simulink model "acc_with_sensor_copy"  (R2021b)
settings: Solver=FixedStepAuto  StartTime=0.0  StopTime=206  FixedStep=0.0005  RelTol=1e-3
InitFcn:
  | G=9.81;
  | m=1660;
  | rw=0.325;
  | Caf=74070;
  | Car=58525;
  | Iz=2778.5;
  | d = 1.502;
  | lf =1.1135;
  | lr =1.5065;
  | L = 2.62;
  | kph2mps=1/3.6;
values from neighbouring files (symbols this model uses):
  Leftdis_PV_switch = 2    [acc_plot_backup.m]
  s_path = [0 1.10508939428 2.2141958029 3.32141571172 4.42705301151 5.53154548532 6.63517443471 7.73808041313 8.84055018688 9.94289959674 11.0453539299 12.1480581097 ... (1001 elements, 1001x1)]    [200_100radius.mat]    (also in LV_Clothoid_S_Turn_path.mat = [0 0.966832089581 1.93621320584 2.90214024471 3.86476766313 ; NEDC_path.mat = [0 0.414605943146 0.832514087334 1.25401518562 1.68216660344; Straight_East_into_curve.mat = [0 1.65770560069 3.32192925577 4.98420060507 6.64484613518 8; acc_plot_backup.m = Station_HV_m)
  X_path = [0 1.10508939428 2.2141958029 3.32141571172 4.42705301151 5.53154548532 6.63517443471 7.73808041313 8.84055018688 9.94289959674 11.0453539299 12.1480581097 ... (1001 elements, 1001x1)]    [200_100radius.mat]    (also in LV_Clothoid_S_Turn_path.mat = [-10 -9.03316791042 -8.06378679416 -7.09785975529 -6.1352323; NEDC_path.mat = [0 0.414605943146 0.832514087334 1.25401518562 1.68216660344; Straight_East_into_curve.mat = [0 1.65770560069 3.32192925577 4.98420060507 6.64484613518 8; acc_plot_backup.m = X_HV_m)
  Y_path = [0 -1.70364610795e-18 -7.41532896709e-18 1.46822109542e-17 4.74557362791e-17 6.12980216762e-17 9.25043977736e-17 1.24088240159e-16 1.5099156923e-16 1.7058517853e-16 1.90629227614e-16 2.09673434424e-16 ... (1001 elements, 1001x1)]    [200_100radius.mat]    (also in LV_Clothoid_S_Turn_path.mat = [0 -8.46153035536e-19 5.07382551045e-18 2.07356032218e-17 3.; NEDC_path.mat = [0 -3.50680326162e-18 -2.14111304971e-18 3.38197671014e-18 3; Straight_East_into_curve.mat = [0 1.29197709199e-18 2.81882429322e-18 3.49020462564e-17 6.7; acc_plot_backup.m = Y_HV_m)
undefined symbols (not defined in the file or in its folder): C_TICK_TIME_S, Cut_in_Secenary_flg, ENUM_ACCSTATE_DISABLED, ENUM_ACCSTATE_OFF, ENUM_ACCSTATE_STANDBY, FALSE, KVDI_ACCLongPressTime_ms, KVDI_ACCMaxActSpeed_kph, KVDI_ACCSetSpdIntial_kph, KVDI_ACCSpdLargeChange_kph, KVDI_LongPressConTime_ms, ONE_FLOAT, ONE_INT, Path_selector, R, Rw, T, TRUE, UseTTC_switch, ZERO_FLOAT, ZERO_INT
libraries: simulink x15, dspstat3 x4, simulink_extras x2, Solver_SF x1
(part 6 of 8)

== system acc_with_sensor_copy/V_rel Estimation ==
  cut_in_flg : Inport
  a_c : Inport  Port=2
  S_rel : Inport  Port=3
  initial_value : Inport  Port=4
  Add3 : Sum  Inputs=-+
  Delay1 : Delay  DelayLength=1  InitialConditionSource=Input port  SampleTime=0.1
      settings: InputPortMap=u0,p4
  Kalman filter : Subsystem
  sample time : Gain  Gain=1/0.1
  s_rel : Outport
  v_rel : Outport  Port=2
  a_rel : Outport  Port=3
  wires:
  S_rel/1 -> Kalman filter/3(S_rel)
  Kalman filter/1(s_rel) -> s_rel/1
  Add3/1 -> sample time/1
  Delay1/1 -> Add3/1
  a_c/1 -> Delay1/1, Delay1/2, Add3/2
  Kalman filter/2(v_rel) -> v_rel/1
  sample time/1 -> Kalman filter/2(Jerk)  "Jerk"
  Kalman filter/3(a_rel) -> a_rel/1
  initial_value/1 -> Kalman filter/4(initial_value)
  cut_in_flg/1 -> Kalman filter/1(cut_in_flg)

== system acc_with_sensor_copy/acceleration_apr1 ==
  acc_b : Inport
  Abs : Abs
  Constant1 : Constant  Value=0
  Switch : Switch  Criteria=u2 > Threshold  Threshold=0.01
  acc_a : Outport  VectorParamsAs1DForOutWhenUnconnected=off
  wires:
  Switch/1 -> acc_a/1
  acc_b/1 -> Abs/1, Switch/1
  Constant1/1 -> Switch/3
  Abs/1 -> Switch/2

== system acc_with_sensor_copy/acceleration_apr4 ==
  acc_b : Inport
  Abs : Abs
  Constant1 : Constant  Value=0
  Switch : Switch  Criteria=u2 > Threshold  Threshold=0.01
  acc_a : Outport  VectorParamsAs1DForOutWhenUnconnected=off
  wires:
  Abs/1 -> Switch/2
  Constant1/1 -> Switch/3
  acc_b/1 -> Switch/1, Abs/1
  Switch/1 -> acc_a/1

== system acc_with_sensor_copy/cmd_limiter1 ==
  ax_cmd : Inport
  Constant : Constant  Value=0.1  SampleTime=0.1
  Constant1 : Constant  Value=2.5  SampleTime=0.1
  Constant2 : Constant  Value=-2.5  SampleTime=0.1
  Saturation : Saturate  UpperLimit=2  LowerLimit=-2
  rate_limit : Subsystem
  ax_cmd1 : Outport
  wires:
  Constant2/1 -> rate_limit/4(ratelimt_decps)
  Constant1/1 -> rate_limit/3(ratelimt_incps)
  ax_cmd/1 -> Saturation/1
  Constant/1 -> rate_limit/2(Sample_Time)
  rate_limit/1(ax_cmd1) -> ax_cmd1/1
  Saturation/1 -> rate_limit/1(input_raw)

== system acc_with_sensor_copy/cmd_limiter4 ==
  ax_cmd : Inport
  Constant : Constant  Value=0.1  SampleTime=0.1
  Constant1 : Constant  Value=2.5  SampleTime=0.1
  Constant2 : Constant  Value=-2.5  SampleTime=0.1
  Saturation : Saturate  UpperLimit=2  LowerLimit=-2
  rate_limit : Subsystem
  ax_cmd1 : Outport
  wires:
  rate_limit/1(ax_cmd1) -> ax_cmd1/1
  Constant/1 -> rate_limit/2(Sample_Time)
  ax_cmd/1 -> Saturation/1
  Constant1/1 -> rate_limit/3(ratelimt_incps)
  Constant2/1 -> rate_limit/4(ratelimt_decps)
  Saturation/1 -> rate_limit/1(input_raw)

== system acc_with_sensor_copy/divide ==
  dividend : Inport
  divisor : Inport  Port=2
  default_value : Inport  Port=3
  Divide : Product  Inputs=*/
  Interval Test : simulink/Logic and Bit Operations/Interval Test  IntervalClosedRight=on  uplimit=5/3.6  IntervalClosedLeft=on  lowlimit=-1  OutDataTypeStr=boolean
  Logical Operator : Logic  Operator=NOT  Inputs=1  AllPortsSameDT=off  OutDataTypeStr=boolean
  Scope : Scope
  Switch : Switch  Criteria=u2 ~= 0  Threshold=0.5
  quotient : Outport
  wires:
  Logical Operator/1 -> Switch/2
  default_value/1 -> Switch/3  "default_value"
  Interval Test/1 -> Scope/1, Logical Operator/1
  Switch/1 -> quotient/1
  Divide/1 -> Switch/1
  divisor/1 -> Interval Test/1, Divide/2  "divisor"
  dividend/1 -> Divide/1  "dividend"

== system acc_with_sensor_copy/divide1 ==
  dividend : Inport
  divisor : Inport  Port=2
  default_value : Inport  Port=3
  Divide : Product  Inputs=*/
  Interval Test : simulink/Logic and Bit Operations/Interval Test  IntervalClosedRight=on  uplimit=1  IntervalClosedLeft=on  lowlimit=-1  OutDataTypeStr=boolean
  Logical Operator : Logic  Operator=NOT  Inputs=1  AllPortsSameDT=off  OutDataTypeStr=boolean
  Scope : Scope
  Switch : Switch  Criteria=u2 ~= 0  Threshold=0.5
  quotient : Outport
  wires:
  Logical Operator/1 -> Switch/2
  default_value/1 -> Switch/3  "default_value"
  Interval Test/1 -> Scope/1, Logical Operator/1
  Switch/1 -> quotient/1
  Divide/1 -> Switch/1
  divisor/1 -> Interval Test/1, Divide/2  "divisor"
  dividend/1 -> Divide/1  "dividend"

== system acc_with_sensor_copy/divide2 ==
  dividend : Inport
  divisor : Inport  Port=2
  default_value : Inport  Port=3
  Divide : Product  Inputs=*/
  Interval Test : simulink/Logic and Bit Operations/Interval Test  IntervalClosedRight=on  uplimit=15/3.6  IntervalClosedLeft=on  lowlimit=-1  OutDataTypeStr=boolean
  Logical Operator : Logic  Operator=NOT  Inputs=1  AllPortsSameDT=off  OutDataTypeStr=boolean
  Scope : Scope
  Switch : Switch  Criteria=u2 ~= 0  Threshold=0.5
  quotient : Outport
  wires:
  dividend/1 -> Divide/1  "dividend"
  divisor/1 -> Divide/2, Interval Test/1  "divisor"
  Divide/1 -> Switch/1
  Switch/1 -> quotient/1
  Interval Test/1 -> Logical Operator/1, Scope/1
  default_value/1 -> Switch/3  "default_value"
  Logical Operator/1 -> Switch/2

== system acc_with_sensor_copy/divide3 ==
  dividend : Inport
  divisor : Inport  Port=2
  default_value : Inport  Port=3
  Divide : Product  Inputs=*/
  Interval Test : simulink/Logic and Bit Operations/Interval Test  IntervalClosedRight=on  uplimit=-0.1  IntervalClosedLeft=on  lowlimit=-inf  OutDataTypeStr=boolean
  Logical Operator : Logic  Operator=NOT  Inputs=1  AllPortsSameDT=off  OutDataTypeStr=boolean
  Scope : Scope
  Switch : Switch  Criteria=u2 ~= 0  Threshold=0.5
  quotient : Outport
  wires:
  dividend/1 -> Divide/1  "dividend"
  divisor/1 -> Divide/2, Interval Test/1  "divisor"
  Divide/1 -> Switch/1
  Switch/1 -> quotient/1
  Interval Test/1 -> Logical Operator/1, Scope/1
  default_value/1 -> Switch/3  "default_value"
  Logical Operator/1 -> Switch/2

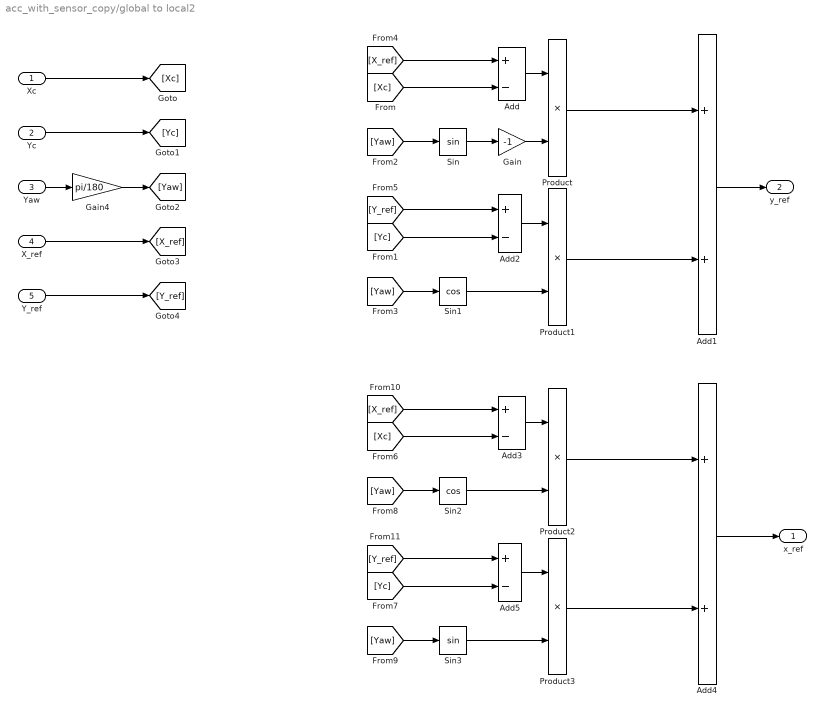
== system acc_with_sensor_copy/global to local2 ==
  Xc : Inport
  Yc : Inport  Port=2
  Yaw : Inport  Port=3
  X_ref : Inport  Port=4
  Y_ref : Inport  Port=5
  Add{,2..3,5} (4 alike) : Sum  Inputs=+-
  Add1 : Sum
  Add4 : Sum
  Gain : Gain  Gain=-1
  Gain4 : Gain  Gain=pi/180
  Product{,1..3} (4 alike) : Product
  Sin : Trigonometry
  Sin1 : Trigonometry  Operator=cos
  Sin2 : Trigonometry  Operator=cos
  Sin3 : Trigonometry
  x_ref : Outport
  y_ref : Outport  Port=2
  wires:
  [X_ref] -> Add3/1
  [Y_ref] -> Add5/1
  Sin2/1 -> Product2/2
  Add3/1 -> Product2/1
  Product2/1 -> Add4/1
  Sin3/1 -> Product3/2
  Add5/1 -> Product3/1
  Product3/1 -> Add4/2
  Add4/1 -> x_ref/1
  [Yaw] -> Sin2/1
  [Yc] -> Add5/2
  [Xc] -> Add3/2
  [Yaw] -> Sin3/1
  Gain4/1 -> [Yaw]
  Y_ref/1 -> [Y_ref]
  X_ref/1 -> [X_ref]
  [Yaw] -> Sin1/1
  Yaw/1 -> Gain4/1
  Yc/1 -> [Yc]
  Xc/1 -> [Xc]
  [Xc] -> Add/2
  [Yc] -> Add2/2
  [Yaw] -> Sin/1
  Add1/1 -> y_ref/1
  Product1/1 -> Add1/2
  Add2/1 -> Product1/1
  Sin1/1 -> Product1/2
  Product/1 -> Add1/1
  Add/1 -> Product/1
  Gain/1 -> Product/2
  Sin/1 -> Gain/1
  [Y_ref] -> Add2/1
  [X_ref] -> Add/1

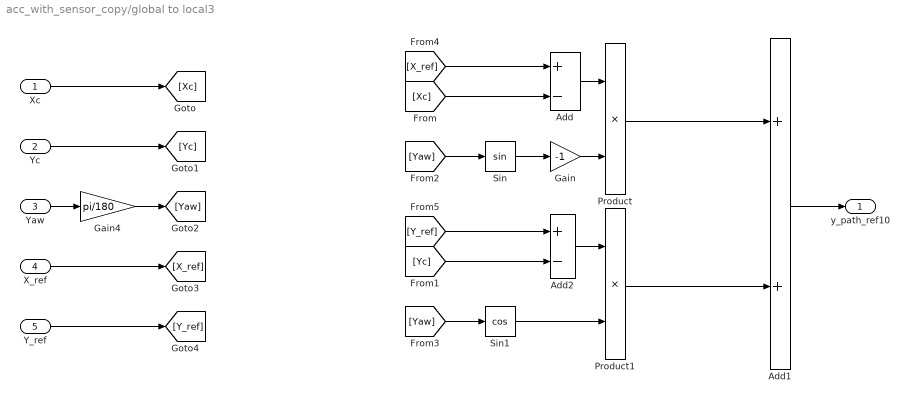
== system acc_with_sensor_copy/global to local3 ==
  Xc : Inport
  Yc : Inport  Port=2
  Yaw : Inport  Port=3
  X_ref : Inport  Port=4
  Y_ref : Inport  Port=5
  Add : Sum  Inputs=+-
  Add1 : Sum
  Add2 : Sum  Inputs=+-
  Gain : Gain  Gain=-1
  Gain4 : Gain  Gain=pi/180
  Product : Product
  Product1 : Product
  Sin : Trigonometry
  Sin1 : Trigonometry  Operator=cos
  y_path_ref10 : Outport
  wires:
  Gain4/1 -> [Yaw]
  Y_ref/1 -> [Y_ref]
  X_ref/1 -> [X_ref]
  [Yaw] -> Sin1/1
  Yaw/1 -> Gain4/1
  Yc/1 -> [Yc]
  Xc/1 -> [Xc]
  [Xc] -> Add/2
  [Yc] -> Add2/2
  [Yaw] -> Sin/1
  Add1/1 -> y_path_ref10/1
  Product1/1 -> Add1/2
  Add2/1 -> Product1/1
  Sin1/1 -> Product1/2
  Product/1 -> Add1/1
  Add/1 -> Product/1
  Gain/1 -> Product/2
  Sin/1 -> Gain/1
  [Y_ref] -> Add2/1
  [X_ref] -> Add/1

== system acc_with_sensor_copy/preview ==
  In1 : Inport
  In2 : Inport  Port=2
  Add9 : Sum
  Constant20 : Constant  Value=s_path
  Constant21 : Constant  Value=X_path
  Constant22 : Constant  Value=s_path
  Constant23 : Constant  Value=Y_path
  Constant49 : Constant  Value=[1:10]'
  Constant51 : Constant  Value=0.1
  Demux4 : Demux  Outputs=[1 9]
  Demux5 : Demux  Outputs=[1 9]
  Lookup Table Dynamic : simulink/Lookup Tables/Lookup Table Dynamic  LookUpMeth=Interpolation-Use End Values  OutDataType=fixdt('double')  OutScaling=[]  OutputDataTypeScalingMode=Specify via dialog  OutDataTypeStr=double  DoSatur=off
  Lookup Table Dynamic1 : simulink/Lookup Tables/Lookup Table Dynamic  LookUpMeth=Interpolation-Use End Values  OutDataType=fixdt('double')  OutScaling=[]  OutputDataTypeScalingMode=Specify via dialog  OutDataTypeStr=double  DoSatur=off
  Product1 : Product
  Product10 : Product
  Scope7 : Scope
  Terminator : Terminator
  Terminator1 : Terminator
  To Workspace27 : ToWorkspace  VariableName=X_ref  SampleTime=-1
  To Workspace28 : ToWorkspace  VariableName=Y_ref  SampleTime=-1
  X_ref : Outport
  Y_ref : Outport  Port=2
  wires:
  Constant23/1 -> Lookup Table Dynamic1/3
  Product10/1 -> Add9/2
  Product1/1 -> Product10/2
  Constant22/1 -> Lookup Table Dynamic1/2
  Constant20/1 -> Lookup Table Dynamic/2
  Constant21/1 -> Lookup Table Dynamic/3
  Lookup Table Dynamic1/1 -> Y_ref/1, Demux5/1
  Demux5/1 -> To Workspace28/1
  In1/1 -> Add9/1
  Lookup Table Dynamic/1 -> X_ref/1, Demux4/1
  In2/1 -> Product10/1
  Constant51/1 -> Product1/2
  Add9/1 -> Lookup Table Dynamic1/1, Scope7/1, Lookup Table Dynamic/1
  Constant49/1 -> Product1/1
  Demux4/1 -> To Workspace27/1
  Demux5/2 -> Terminator1/1
  Demux4/2 -> Terminator/1

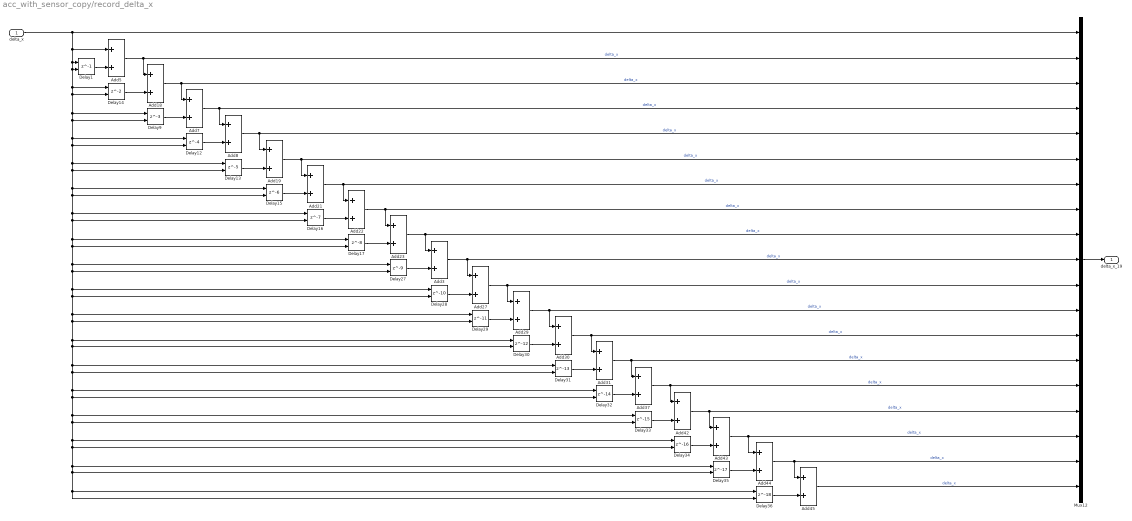
== system acc_with_sensor_copy/record_delta_x ==
  delta_x : Inport
  Add{3,5,7..8,18..19,21..23,27,29..31,37,42..45} (18 alike) : Sum
  Delay1 : Delay  DelayLength=1  InitialConditionSource=Input port
      settings: InputPortMap=u0,p4
  Delay12 : Delay  DelayLength=4  InitialConditionSource=Input port
      settings: InputPortMap=u0,p4
  Delay13 : Delay  DelayLength=5  InitialConditionSource=Input port
      settings: InputPortMap=u0,p4
  Delay14 : Delay  InitialConditionSource=Input port
      settings: InputPortMap=u0,p4
  Delay15 : Delay  DelayLength=6  InitialConditionSource=Input port
      settings: InputPortMap=u0,p4
  Delay16 : Delay  DelayLength=7  InitialConditionSource=Input port
      settings: InputPortMap=u0,p4
  Delay17 : Delay  DelayLength=8  InitialConditionSource=Input port
      settings: InputPortMap=u0,p4
  Delay27 : Delay  DelayLength=9  InitialConditionSource=Input port
      settings: InputPortMap=u0,p4
  Delay28 : Delay  DelayLength=10  InitialConditionSource=Input port
      settings: InputPortMap=u0,p4
  Delay29 : Delay  DelayLength=11  InitialConditionSource=Input port
      settings: InputPortMap=u0,p4
  Delay30 : Delay  DelayLength=12  InitialConditionSource=Input port
      settings: InputPortMap=u0,p4
  Delay31 : Delay  DelayLength=13  InitialConditionSource=Input port
      settings: InputPortMap=u0,p4
  Delay32 : Delay  DelayLength=14  InitialConditionSource=Input port
      settings: InputPortMap=u0,p4
  Delay33 : Delay  DelayLength=15  InitialConditionSource=Input port
      settings: InputPortMap=u0,p4
  Delay34 : Delay  DelayLength=16  InitialConditionSource=Input port
      settings: InputPortMap=u0,p4
  Delay35 : Delay  DelayLength=17  InitialConditionSource=Input port
      settings: InputPortMap=u0,p4
  Delay36 : Delay  DelayLength=18  InitialConditionSource=Input port
      settings: InputPortMap=u0,p4
  Delay9 : Delay  DelayLength=3  InitialConditionSource=Input port
      settings: InputPortMap=u0,p4
  Mux12 : Mux  Inputs=19
  delta_x_19 : Outport
  wires:
  Add19/1 -> Mux12/6, Add21/1  "delta_x"
  Delay13/1 -> Add19/2
  Add44/1 -> Add45/1, Mux12/18  "delta_x"
  delta_x/1 -> Mux12/1, Delay14/2, Delay9/1, Delay15/1, Delay27/2, Delay28/1, Delay30/2, Delay31/1, Delay32/1, Delay33/1, Delay33/2, Delay34/1, Delay35/1, Delay36/1, Delay36/2, Delay35/2, Delay34/2, Delay32/2, Delay31/2, Delay30/1, Delay29/2, Delay29/1, Delay28/2, Delay27/1, Delay17/2, Delay17/1, Delay16/2, Delay16/1, Delay15/2, Delay13/2, Delay13/1, Delay12/2, Delay12/1, Delay9/2, Delay14/1, Delay1/2, Delay1/1, Add5/1
  Add29/1 -> Mux12/12, Add30/1  "delta_x"
  Add5/1 -> Mux12/2, Add18/1  "delta_x"
  Add18/1 -> Mux12/3, Add7/1  "delta_x"
  Delay29/1 -> Add29/2
  Delay1/1 -> Add5/2
  Add31/1 -> Mux12/14, Add37/1  "delta_x"
  Delay33/1 -> Add42/2
  Add23/1 -> Mux12/9, Add3/1  "delta_x"
  Delay9/1 -> Add7/2
  Add42/1 -> Add43/1, Mux12/16  "delta_x"
  Mux12/1 -> delta_x_19/1
  Delay14/1 -> Add18/2
  Add21/1 -> Mux12/7, Add22/1  "delta_x"
  Add30/1 -> Mux12/13, Add31/1  "delta_x"
  Delay34/1 -> Add43/2
  Delay17/1 -> Add23/2
  Delay27/1 -> Add3/2
  Add45/1 -> Mux12/19  "delta_x"
  Delay31/1 -> Add31/2
  Add43/1 -> Add44/1, Mux12/17  "delta_x"
  Delay15/1 -> Add21/2
  Add8/1 -> Mux12/5, Add19/1  "delta_x"
  Delay32/1 -> Add37/2
  Delay35/1 -> Add44/2
  Delay36/1 -> Add45/2
  Add27/1 -> Mux12/11, Add29/1  "delta_x"
  Add3/1 -> Mux12/10, Add27/1  "delta_x"
  Delay28/1 -> Add27/2
  Delay16/1 -> Add22/2
  Add22/1 -> Mux12/8, Add23/1  "delta_x"
  Delay30/1 -> Add30/2
  Add37/1 -> Mux12/15, Add42/1  "delta_x"
  Delay12/1 -> Add8/2
  Add7/1 -> Mux12/4, Add8/1  "delta_x"

== system acc_with_sensor_copy/record_delta_yaw ==
  delta_yaw : Inport
  Add78 : Sum  Inputs=+-
  Delay68 : Delay  DelayLength=1  InitialConditionSource=Input port
      settings: InputPortMap=u0,p4
  Delay69 : Delay  InitialConditionSource=Input port
      settings: InputPortMap=u0,p4
  Delay70 : Delay  DelayLength=3  InitialConditionSource=Input port
      settings: InputPortMap=u0,p4
  Delay71 : Delay  DelayLength=4  InitialConditionSource=Input port
      settings: InputPortMap=u0,p4
  Delay72 : Delay  DelayLength=5  InitialConditionSource=Input port
      settings: InputPortMap=u0,p4
  Delay73 : Delay  DelayLength=6  InitialConditionSource=Input port
      settings: InputPortMap=u0,p4
  Delay74 : Delay  DelayLength=7  InitialConditionSource=Input port
      settings: InputPortMap=u0,p4
  Delay75 : Delay  DelayLength=8  InitialConditionSource=Input port
      settings: InputPortMap=u0,p4
  Delay76 : Delay  DelayLength=9  InitialConditionSource=Input port
      settings: InputPortMap=u0,p4
  Delay77 : Delay  DelayLength=10  InitialConditionSource=Input port
      settings: InputPortMap=u0,p4
  Delay78 : Delay  DelayLength=11  InitialConditionSource=Input port
      settings: InputPortMap=u0,p4
  Delay79 : Delay  DelayLength=12  InitialConditionSource=Input port
      settings: InputPortMap=u0,p4
  Delay80 : Delay  DelayLength=13  InitialConditionSource=Input port
      settings: InputPortMap=u0,p4
  Delay81 : Delay  DelayLength=14  InitialConditionSource=Input port
      settings: InputPortMap=u0,p4
  Delay82 : Delay  DelayLength=15  InitialConditionSource=Input port
      settings: InputPortMap=u0,p4
  Delay83 : Delay  DelayLength=16  InitialConditionSource=Input port
      settings: InputPortMap=u0,p4
  Delay84 : Delay  DelayLength=17  InitialConditionSource=Input port
      settings: InputPortMap=u0,p4
  Delay85 : Delay  DelayLength=18  InitialConditionSource=Input port
      settings: InputPortMap=u0,p4
  Delay86 : Delay  DelayLength=19  InitialConditionSource=Input port
      settings: InputPortMap=u0,p4
  Mux18 : Mux  Inputs=19
  delta_yaw_19 : Outport
  wires:
  Delay84/1 -> Mux18/17
  Delay72/1 -> Mux18/5
  Delay73/1 -> Mux18/6
  Delay78/1 -> Mux18/11
  Delay71/1 -> Mux18/4
  Delay68/1 -> Mux18/1
  Delay76/1 -> Mux18/9
  delta_yaw/1 -> Delay68/1, Delay68/2, Delay86/2, Delay86/1, Delay85/2, Delay85/1, Delay84/2, Delay84/1, Delay83/2, Delay83/1, Delay82/2, Delay82/1, Delay81/2, Delay81/1, Delay80/2, Delay80/1, Delay79/2, Delay79/1, Delay78/2, Delay78/1, Delay77/2, Delay77/1, Delay76/2, Delay76/1, Delay75/2, Delay75/1, Delay74/2, Delay74/1, Delay73/2, Delay73/1, Delay72/2, Delay72/1, Delay71/2, Delay71/1, Delay70/2, Delay70/1, Delay69/2, Delay69/1, Add78/1
  Delay81/1 -> Mux18/14
  Delay75/1 -> Mux18/8
  Delay80/1 -> Mux18/13
  Delay86/1 -> Mux18/19
  Delay82/1 -> Mux18/15
  Delay69/1 -> Mux18/2
  Delay70/1 -> Mux18/3
  Delay74/1 -> Mux18/7
  Mux18/1 -> Add78/2
  Delay77/1 -> Mux18/10
  Add78/1 -> delta_yaw_19/1
  Delay85/1 -> Mux18/18
  Delay79/1 -> Mux18/12
  Delay83/1 -> Mux18/16

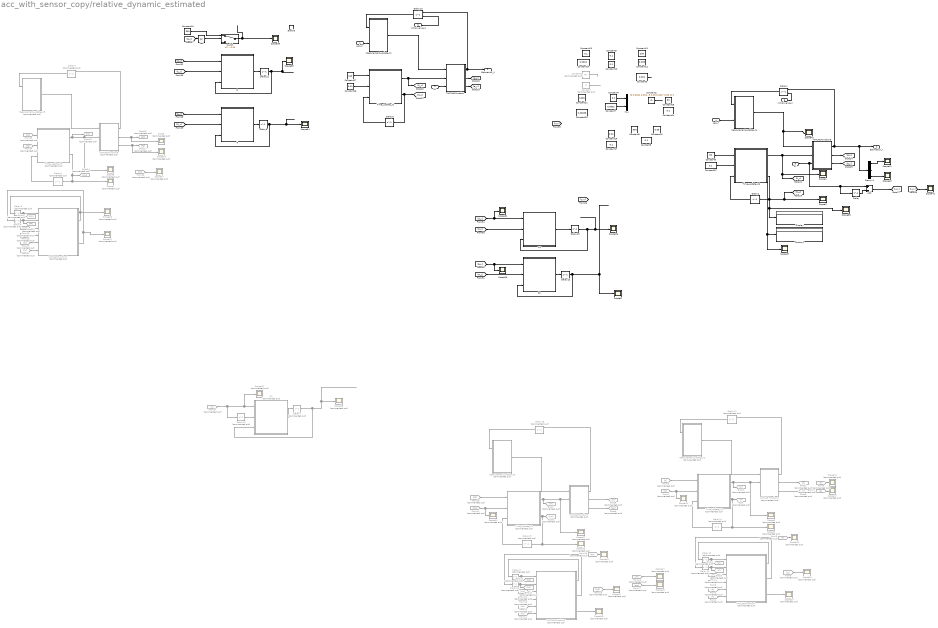
== system acc_with_sensor_copy/relative_dynamic_estimated ==
  Jerk_X : Inport
  RX : Inport  Port=2
  Initial_value_X : Inport  Port=3
  Jerk_Y : Inport  Port=4
  RY : Inport  Port=5
  Initial_value_Y : Inport  Port=6
  Enable : EnablePort
  Abs : Abs
  Add : Sum  Inputs=+-
  Constant : Constant  Commented=on  Value=R
  Constant1 : Constant  Commented=on  Value=Rw
  Constant{4..5,9..10,13,17,22,24} (8 alike) : Constant  Value=0.1
  Constant11 : Constant  Value=200
  Constant12 : Constant  Value=0.005
  Constant14 : Constant  Value=0.0001
  Constant15 : Constant  Value=0.05
  Constant16 : Constant  Value=300
  Constant19 : Constant  Value=0.01
  Constant2 : Constant  Value=[0 0.0001 0.0017;0.0001 0.0025 0.05;0.0017 0.05 1]*1
  Constant20 : Constant  Value=0.00005
  Constant21 : Constant  Value=1000
  Constant25 : Constant  Value=50
  Constant26 : Constant  Value=0.01
  Constant27 : Constant  Value=100
  Constant3 : Constant  Value=0.001
  Constant6 : Constant  Value=50
  Constant7 : Constant  Value=0.0001
  Constant8 : Constant  Value=500
  Delay : Delay  DelayLength=1
  Delay1 : Delay  DelayLength=1  InitialConditionSource=Input port  InitialCondition=[0;0;0]  SampleTime=T
      settings: InputPortMap=u0,p4
  Delay10 : Delay  DelayLength=1  InitialConditionSource=Input port  InitialCondition=[0;0;0]  SampleTime=T
      settings: InputPortMap=u0,p4
  Delay11 : Delay  Commented=on  DelayLength=1  InitialConditionSource=Input port  InitialCondition=[0;0;0]  SampleTime=T
      settings: InputPortMap=u0,p4
  Delay12 : Delay  Commented=on  DelayLength=1  InitialCondition=[0 0 0;0 0 0.004;0 0.004 0.8]*0.001  SampleTime=T
  Delay13 : Delay  Commented=on  DelayLength=1  InitialCondition=0.001  SampleTime=T
  Delay14 : Delay  Commented=on  DelayLength=1  InitialCondition=[1 0 0;0 1 0;0 0 1]  SampleTime=T
  Delay15 : Delay  Commented=on  DelayLength=1  InitialConditionSource=Input port  InitialCondition=[0;0;0]  SampleTime=T
      settings: InputPortMap=u0,p4
  Delay16 : Delay  Commented=on  DelayLength=1  InitialCondition=0
  Delay17 : Delay  Commented=on  DelayLength=1  InitialCondition=[0 0 0;0 0 0.004;0 0.004 0.8]*0.01  SampleTime=T
  Delay18 : Delay  Commented=on  DelayLength=1  InitialCondition=0.001  SampleTime=T
  Delay19 : Delay  Commented=on  DelayLength=1  InitialCondition=[1 0 0;0 1 0;0 0 1]  SampleTime=T
  Delay2 : Delay  DelayLength=1  InitialCondition=[1 0 0;0 1 0;0 0 1]  SampleTime=T
  Delay21 : Delay  DelayLength=1  InitialCondition=[0 0.0001 0.0017;0.0001 0.0025 0.05;0.0017 0.05 1]
  Delay22 : Delay  DelayLength=1  InitialCondition=0.001
  Delay23 : Delay  DelayLength=1  InitialCondition=[0 0.0001 0.0017;0.0001 0.0025 0.05;0.0017 0.05 1]*1e-5
  Delay3 : Delay  Commented=on  DelayLength=1  InitialCondition=[0 0 0;0 0 0.003;0 0.003 0.005]  SampleTime=T
  Delay4 : Delay  Commented=on  DelayLength=1  InitialConditionSource=Input port  InitialCondition=[0;0;0]  SampleTime=T
      settings: InputPortMap=u0,p4
  Delay5 : Delay  Commented=on  DelayLength=1  InitialCondition=0.001  SampleTime=T
  Delay6 : Delay  Commented=on  DelayLength=1  InitialCondition=[1 0 0;0 1 0;0 0 1]  SampleTime=T
  Delay7 : Delay  Commented=on  DelayLength=1  InitialCondition=0.1
  Delay8 : Delay  DelayLength=1  InitialCondition=0.1
  Delay9 : Delay  DelayLength=1  InitialCondition=[1 0 0;0 1 0;0 0 1]  SampleTime=T
  Demux1 : Demux  Outputs=3
  Display : Display
  Display1 : Display
  From : From  Commented=on  GotoTag=M
  From1 : From  Commented=on  GotoTag=K
  From10 : From  Commented=on  GotoTag=MM
  From11 : From  Commented=on  GotoTag=KK
  From12 : From  Commented=on  GotoTag=dd
  From13 : From  Commented=on  GotoTag=ee
  From14 : From  Commented=on  GotoTag=QQ
  From15 : From  Commented=on  GotoTag=RR
  From16 : From  Commented=on  GotoTag=dd
  From17 : From  Commented=on  GotoTag=ee
  From18 : From  Commented=on  GotoTag=RR
  From19 : From  Commented=on  GotoTag=QQ
  From2 : From  Commented=on  GotoTag=d
  From20 : From  Commented=on  GotoTag=MM
  From21 : From  Commented=on  GotoTag=KK
  From22 : From  Commented=on  GotoTag=dd
  From23 : From  Commented=on  GotoTag=ee
  From24 : From  Commented=on  GotoTag=QQ
  From25 : From  Commented=on  GotoTag=RR
  From26 : From  Commented=on  GotoTag=KK
  From27 : From  Commented=on  GotoTag=d
  From3 : From  Commented=on  GotoTag=e
  From4 : From  Commented=on  GotoTag=Q
  From5 : From  Commented=on  GotoTag=R
  From6 : From  Commented=on  GotoTag=d
  From7 : From  Commented=on  GotoTag=e
  From8 : From  Commented=on  GotoTag=R
  From9 : From  Commented=on  GotoTag=Q
  Goto : Goto  Commented=on  GotoTag=M
  Goto1 : Goto  Commented=on  GotoTag=K
  Goto10 : Goto  Commented=on  GotoTag=QQ
  Goto11 : Goto  Commented=on  GotoTag=RR
  Goto12 : Goto  Commented=on  GotoTag=QQ
  Goto13 : Goto  Commented=on  GotoTag=RR
  Goto14 : Goto  Commented=on  GotoTag=MM
  Goto15 : Goto  Commented=on  GotoTag=KK
  Goto16 : Goto  Commented=on  GotoTag=dd
  Goto17 : Goto  Commented=on  GotoTag=ee
  Goto2 : Goto  Commented=on  GotoTag=d
  Goto3 : Goto  Commented=on  GotoTag=e
  Goto4 : Goto  Commented=on  GotoTag=Q
  Goto5 : Goto  Commented=on  GotoTag=R
  Goto6 : Goto  Commented=on  GotoTag=MM
  Goto7 : Goto  Commented=on  GotoTag=KK
  Goto8 : Goto  Commented=on  GotoTag=dd
  Goto9 : Goto  Commented=on  GotoTag=ee
  MATLAB Function : MATLAB Function  TreatAsAtomicUnit=on
  MATLAB Function1 : MATLAB Function  Commented=on  TreatAsAtomicUnit=on
  MATLAB Function2 : MATLAB Function  Commented=on  TreatAsAtomicUnit=on
  MATLAB Function3 : MATLAB Function  Commented=on  TreatAsAtomicUnit=on
  MATLAB Function4 : MATLAB Function  Commented=on  TreatAsAtomicUnit=on
  MATLAB Function5 : MATLAB Function  TreatAsAtomicUnit=on
  MATLAB Function6 : MATLAB Function  Commented=on  TreatAsAtomicUnit=on
  MATLAB Function7 : MATLAB Function  Commented=on  TreatAsAtomicUnit=on
  Measurement_update_X1 : MATLAB Function  TreatAsAtomicUnit=on
  Measurement_update_X2 : MATLAB Function  Commented=on  TreatAsAtomicUnit=on
  Measurement_update_X3 : MATLAB Function  Commented=on  TreatAsAtomicUnit=on
  Measurement_update_X4 : MATLAB Function  TreatAsAtomicUnit=on
  Measurement_update_X5 : MATLAB Function  Commented=on  TreatAsAtomicUnit=on
  Mux : Mux  Inputs=2
  Q : MATLAB Function  TreatAsAtomicUnit=on
  Q1 : MATLAB Function  Commented=on  TreatAsAtomicUnit=on
  Q2 : MATLAB Function  TreatAsAtomicUnit=on
  R : MATLAB Function  TreatAsAtomicUnit=on
  R2 : MATLAB Function  TreatAsAtomicUnit=on
  Scope{,6..28,30} (25 alike) : Scope  Commented=on
  Scope{1..2,5,29,31,34..43} (15 alike) : Scope
  Switch : Switch  Criteria=u2 > Threshold  Threshold=0.04
  Time_update_X1 : MATLAB Function  TreatAsAtomicUnit=on
  Time_update_X2 : MATLAB Function  Commented=on  TreatAsAtomicUnit=on
  Time_update_X3 : MATLAB Function  Commented=on  TreatAsAtomicUnit=on
  Time_update_X5 : MATLAB Function  Commented=on  TreatAsAtomicUnit=on
  Time_update_X6 : MATLAB Function  TreatAsAtomicUnit=on
  Estimation_X : Outport  VectorParamsAs1DForOutWhenUnconnected=off
  Estimation_Y : Outport  Port=2  VectorParamsAs1DForOutWhenUnconnected=off
  wires:
  MATLAB Function/3(e) -> [e_x]
  MATLAB Function/2(d) -> [d_x]
  Constant27/1 -> Time_update_X1/1(Q)
  Constant26/1 -> Time_update_X1/2(R)
  Abs/1 -> Switch/2
  [d_x] -> Abs/1
  Constant16/1 -> Switch/1
  Switch/1 -> Scope39/1
  Constant22/1 -> Time_update_X6/2(R)
  Constant6/1 -> Time_update_X6/1(Q)
  Demux1/3 -> Scope43/1
  Demux1/1 -> Scope42/1
  [yyy] -> Scope41/1
  Delay/1 -> Add/2
  Add/1 -> [yyy]
  Delay22/1 -> Scope5/1, R2/3(R1)
  Constant7/1 -> Mux/2
  Constant4/1 -> Mux/1
  Demux1/2 -> ?
  Delay23/1 -> Scope36/1, Q2/3(Q1)
  Time_update_X6/2(P) -> Display1/1, Scope37/1
  Constant3/1 -> ?
  Constant2/1 -> ?
  Q2/1(Q) -> Delay23/1
  Constant1/1 -> ?
  Constant/1 -> ?
  MATLAB Function5/3(e) -> [e_y]
  MATLAB Function5/2(d) -> [d_y]
  [d_y] -> Q2/1(d), Scope31/1
  [K_y] -> Q2/2(K)
  R2/1(R) -> Delay22/1
  [M_y] -> R2/2(M)
  [e_y] -> R2/1(e), Scope29/1
  Q1/1(Rw) -> Delay7/1
  From27/1 -> Q1/1(d), Scope30/1, Delay16/1
  Delay7/1 -> Scope28/1, Q1/3(Rw1)
  Delay16/1 -> Q1/2(dx)
  Delay21/1 -> Q/3(Q1), Scope35/1
  Q/1(Q) -> Delay21/1
  [K_x] -> Q/2(K)
  [d_x] -> Q/1(d)
  [M_x] -> R/2(M)
  R/1(R) -> Delay8/1
  [e_x] -> R/1(e)
  Delay8/1 -> R/3(R1), Scope34/1
  RX/1 -> MATLAB Function/3(y)
  From26/1 -> Scope27/1
  Initial_value_X/1 -> Delay10/2
  Delay4/1 -> Measurement_update_X5/1(X_e)
  MATLAB Function6/1(X_e) -> Delay4/1
  Measurement_update_X5/1(X_b) -> MATLAB Function6/1(X_b)
  Time_update_X5/2(M2) -> Scope7/1, Delay6/1, Goto14/1
  From22/1 -> MATLAB Function7/5(d)
  Delay6/1 -> Time_update_X5/3(M)
  Time_update_X5/1(K) -> MATLAB Function6/2(K), Scope6/1, Goto15/1
  From21/1 -> MATLAB Function7/6(K)
  From20/1 -> MATLAB Function7/3(M)
  MATLAB Function7/2(R2) -> Delay5/1, Scope26/1
  MATLAB Function6/3(e) -> Goto17/1, Scope24/1
  From24/1 -> Time_update_X5/2(Q)
  From25/1 -> Time_update_X5/1(R)
  MATLAB Function7/1(Q2) -> Scope25/1, Delay3/1
  From23/1 -> MATLAB Function7/4(e)
  Delay5/1 -> Goto13/1, MATLAB Function7/2(R)
  Delay3/1 -> Goto12/1, MATLAB Function7/1(Q)
  MATLAB Function6/2(d) -> Goto16/1, Scope/1
  RY/1 -> MATLAB Function5/3(y), Delay/1, Add/1
  Initial_value_Y/1 -> Delay1/2
  Measurement_update_X4/1(X_b) -> MATLAB Function5/1(X_b), Scope40/1
  MATLAB Function5/1(X_e) -> Delay1/1, Estimation_Y/1, Demux1/1
  Delay1/1 -> Measurement_update_X4/1(X_e)
  Time_update_X6/1(K) -> Scope1/1, [K_y], MATLAB Function5/2(K)
  Time_update_X6/3(M2) -> Delay2/1, Scope2/1, [M_y], Display/1, Scope38/1
  Delay2/1 -> Time_update_X6/3(M)
  Jerk_Y/1 -> Measurement_update_X4/2(u)
  Jerk_X/1 -> Measurement_update_X1/2(u)
  MATLAB Function3/2(d) -> Goto8/1
  Delay17/1 -> MATLAB Function4/1(Q), Goto10/1
  Time_update_X3/1(K) -> MATLAB Function3/2(K), Scope22/1, Goto7/1
  From13/1 -> MATLAB Function4/4(e)
  From15/1 -> Time_update_X3/1(R)
  From19/1 -> Scope21/1
  MATLAB Function4/1(Q2) -> Delay17/1
  Delay18/1 -> MATLAB Function4/2(R), Goto11/1
  From10/1 -> MATLAB Function4/3(M)
  MATLAB Function4/2(R2) -> Delay18/1
  Delay15/1 -> Measurement_update_X3/1(X_e)
  From11/1 -> MATLAB Function4/6(K)
  Delay19/1 -> Time_update_X3/3(M)
  From12/1 -> MATLAB Function4/5(d)
  From17/1 -> Scope18/1
  From18/1 -> Scope19/1
  From16/1 -> Scope17/1
  MATLAB Function3/3(e) -> Goto9/1
  Time_update_X3/2(M2) -> Goto6/1, Delay19/1, Scope23/1
  Measurement_update_X3/1(X_b) -> MATLAB Function3/1(X_b)
  From14/1 -> Time_update_X3/2(Q), Scope16/1
  MATLAB Function3/1(X_e) -> Delay15/1
  MATLAB Function4/3(G) -> Scope20/1
  From9/1 -> Scope15/1
  MATLAB Function2/3(G) -> Scope14/1
  From8/1 -> Scope13/1
  From7/1 -> Scope12/1
  From6/1 -> Scope11/1
  From4/1 -> Time_update_X2/2(Q), Scope10/1
  MATLAB Function2/1(Q2) -> Delay12/1
  Time_update_X2/2(M2) -> Goto/1, Delay14/1, Scope9/1
  From1/1 -> MATLAB Function2/6(K)
  Delay13/1 -> MATLAB Function2/2(R), Goto5/1
  Delay14/1 -> Time_update_X2/3(M)
  Time_update_X2/1(K) -> MATLAB Function1/2(K), Scope8/1, Goto1/1
  Delay11/1 -> Measurement_update_X2/1(X_e)
  Measurement_update_X2/1(X_b) -> MATLAB Function1/1(X_b)
  MATLAB Function1/1(X_e) -> Delay11/1
  MATLAB Function1/2(d) -> Goto2/1
  From2/1 -> MATLAB Function2/5(d)
  From5/1 -> Time_update_X2/1(R)
  MATLAB Function1/3(e) -> Goto3/1
  MATLAB Function2/2(R2) -> Delay13/1
  From/1 -> MATLAB Function2/3(M)
  From3/1 -> MATLAB Function2/4(e)
  Delay12/1 -> MATLAB Function2/1(Q), Goto4/1
  MATLAB Function/1(X_e) -> Delay10/1, Estimation_X/1
  Time_update_X1/2(M2) -> Delay9/1, [M_x]
  Measurement_update_X1/1(X_b) -> MATLAB Function/1(X_b)
  Delay9/1 -> Time_update_X1/3(M)
  Delay10/1 -> Measurement_update_X1/1(X_e)
  Time_update_X1/1(K) -> MATLAB Function/2(K), [K_x]

== system acc_with_sensor_copy/rolling_avg ==
  note: new_average = [ (sample_interval)/(sample_interval + time_constant) ] * (new_value - old_ave) + old_ave
  note: - (FK_TMR/TC)
      |                                    f  =  1  -  e
      |
      |       Where "f" is called the filter constant in the difference equation:
      |
      |                    new_average = f * new_value + (1 - f) * old_average
  note: Using the first two terms of the series expansion:
      |
      |                     x                     x2
      |                                e   =  1  +  x  +  --  + ......
      |                                           2!
      |
      |       Simplifying, the exponential "f" becomes:
      |
      |                  - (FK_TMR/TC)              1
      |           f  =  1  -  e                    =  1  -  -------------  =  . . .
      |                                                    (FK_TMR/TC)
      |                           e
      |
      |                              1                      1
      |          f  =  1  -  ---------------------------------  =    ------------------- .
      |                                  1 + (FK_TMR / TC)       1 + (TC / FK_TMR)
  new_value : Inport
  old_ave : Inport  Port=2
  delta_t : Inport  Port=3
  tc : Inport  Port=4
  Divide : Product  Inputs=*/
  IC : UnitDelay  Tag=struct('comment',struct('text','','placement',1),'logdata',struct('maxnumvals',inf,'plotchannels',[],'stepsize',0,'downsampling',1,'loggingmode',3,'channels',1),'output',struct('width',1,'name','$S_$B','unit','','type','Int16','offset',0,'max',NaN,'min',NaN,'freeze',1,'lsb',1,'arb',0,'class','default','address','','description','','autoscalingmode',1,'lowerheadroom',1,'upperheadroom',1,'headroomunit','bit','checkmin',0,'checkmax',0,'show',0,'initial','2'),'state',0,'dt','-1','date',731455.586925799)  InitialCondition=1  SampleTime=0.1  HasFrameUpgradeWarning=on
  Interval Test : simulink/Logic and Bit Operations/Interval Test  IntervalClosedRight=on  uplimit=0.00001  IntervalClosedLeft=on  lowlimit=-0.00001  OutDataTypeStr=boolean
  Logical Operator : Logic  Operator=NOT  AllPortsSameDT=off  OutDataTypeStr=boolean
  Product_tmp1 : Product  Tag=struct('comment',struct('text','','placement',1),'logdata',struct('maxnumvals',inf,'plotchannels',[],'stepsize',0,'downsampling',1,'loggingmode',3,'channels',1),'output',struct('width',1,'name','$S_$B','unit','','type','Int32Bin15','offset',0,'max',65535,'min',-65536,'freeze',1,'lsb',2^-15,'arb',0,'class','default','address','','description','','autoscalingmode',1,'lowerheadroom',1,'upperheadroom',1,'headroomunit','bit','checkmin',0,'checkmax',0,'show',0),'inputs','**','exceptionhandling',1,'date',731455.58640515)  Inputs=**  InputSameDT=on  RndMeth=Zero  OutDataTypeStr=Inherit: Same as first input
  Sum : Sum  Tag=struct('comment',struct('text','','placement',1),'logdata',struct('maxnumvals',inf,'plotchannels',[],'stepsize',0,'downsampling',1,'loggingmode',3,'channels',1),'output',struct('width',1,'name','$S_$B','unit','','type','Int32Bin15','offset',0,'max',65535,'min',-65536,'freeze',1,'lsb',2^-15,'arb',0,'class','default','address','','description','','autoscalingmode',1,'lowerheadroom',1,'upperheadroom',1,'headroomunit','bit','checkmin',0,'checkmax',0,'show',0),'inputs','-+','date',731455.586330463)  Inputs=-+  InputSameDT=on  OutDataTypeStr=Inherit: Same as first input
  Sum1 : Sum  Tag=struct('comment',struct('text','','placement',1),'logdata',struct('maxnumvals',inf,'plotchannels',[],'stepsize',0,'downsampling',1,'loggingmode',3,'channels',1),'output',struct('width',1,'name','$S_$B','unit','','type','Int32Bin15','offset',0,'max',65535,'min',-65536,'freeze',1,'lsb',2^-15,'arb',0,'class','default','address','','description','','autoscalingmode',1,'lowerheadroom',1,'upperheadroom',1,'headroomunit','bit','checkmin',0,'checkmax',0,'show',0),'inputs','++','date',731455.58628235)  InputSameDT=on  OutDataTypeStr=Inherit: Same as first input
  Sum2 : Sum  Tag=struct('comment',struct('text','','placement',1),'logdata',struct('maxnumvals',inf,'plotchannels',[],'stepsize',0,'downsampling',1,'loggingmode',3,'channels',1),'output',struct('width',1,'name','$S_$B','unit','','type','Int32Bin15','offset',0,'max',65535,'min',-65536,'freeze',1,'lsb',2^-15,'arb',0,'class','default','address','','description','','autoscalingmode',1,'lowerheadroom',1,'upperheadroom',1,'headroomunit','bit','checkmin',0,'checkmax',0,'show',0),'inputs','++','date',731455.586506424)  InputSameDT=on  OutDataTypeStr=Inherit: Same as first input
  Switch : Switch  Criteria=u2 ~= 0
  Switch1 : Switch  Tag=struct('comment',struct('text','','placement',1),'logdata',struct('maxnumvals',inf,'plotchannels',[],'stepsize',0,'downsampling',1,'loggingmode',3,'channels',1),'output',struct('width',1,'name','$S_$B','unit','','type','Int32Bin15','offset',0,'max',65535,'min',-65536,'freeze',1,'lsb',2^-15,'arb',0,'class','default','address','','description','','autoscalingmode',1,'lowerheadroom',1,'upperheadroom',1,'headroomunit','bit','checkmin',0,'checkmax',0,'show',0),'threshold',struct('width',1,'name','$S_$B_threshold','unit','','type','Int16','offset',0,'max',NaN,'min',NaN,'freeze',1,'lsb',1,'arb',0,'class','default','address','','description','','value','1','scalar',0),'date',731455.58657044)  Threshold=0.5  InputSameDT=on
  zero : Constant  Tag=struct('comment',struct('text','','placement',1),'output',struct('width',1,'name','$S_$B','unit','','type','Int16','offset',0,'max',NaN,'min',NaN,'freeze',1,'lsb',1,'arb',0,'class','default','address','','description','','value','0','tolerance',1,'show',0),'date',731455.58675544)  Value=0  OutDataTypeStr=Inherit: Inherit via back propagation
  zero1 : Constant  Tag=struct('comment',struct('text','','placement',1),'output',struct('width',1,'name','$S_$B','unit','','type','Int16','offset',0,'max',NaN,'min',NaN,'freeze',1,'lsb',1,'arb',0,'class','default','address','','description','','value','0','tolerance',1,'show',0),'date',731455.58675544)  Value=0  OutDataTypeStr=Inherit: Inherit via back propagation
  new_ave : Outport
  wires:
  Switch/1 -> Sum2/2
  Product_tmp1/1 -> Divide/1
  [new_value] -> Switch1/1
  Sum2/1 -> Switch1/3  "new_ave"
  new_value/1 -> [new_value], Sum/2  "new_value"
  Switch1/1 -> new_ave/1  "new_ave"
  Sum/1 -> Product_tmp1/1
  tc/1 -> Sum1/2
  delta_t/1 -> Sum1/1, Product_tmp1/2  "delta_t"
  zero/1 -> IC/1
  old_ave/1 -> Sum/1, Sum2/1  "old_ave"
  Sum1/1 -> Interval Test/1, Divide/2
  zero1/1 -> Switch/3
  Interval Test/1 -> Logical Operator/1
  Divide/1 -> Switch/1
  Logical Operator/1 -> Switch/2
  IC/1 -> Switch1/2

== system acc_with_sensor_copy/Cut-in strategy/Subsystem8 ==
  TTC : Inport
  Mode : Inport  Port=2
  Constant1 : Constant  Value=0
  Gain : Gain  Gain=5
  Switch : Switch  Criteria=u2 ~= 0
  tau : Outport
  wires:
  Constant1/1 -> Switch/3
  TTC/1 -> Gain/1
  Switch/1 -> tau/1
  Mode/1 -> Switch/2
  Gain/1 -> Switch/1

== system acc_with_sensor_copy/Smooth Switch/Subsystem ==
  TTC : Inport
  Mode : Inport  Port=2
  1-D Lookup Table : Lookup_n-D  NumberOfTableDimensions=1  BreakpointsForDimension1=[0 2 10]  Table=[0.05 0.05 0.5]  InternalRulePriority=Speed  RndMeth=Simplest  InputSameDT=on
  Constant1 : Constant  Value=0.5
  Constant2 : Constant
  Constant3 : Constant  Value=0.01
  Switch : Switch  Criteria=u2 ~= 0
  tau : Outport
  wires:
  Constant1/1 -> Switch/1
  Switch/1 -> tau/1
  Mode/1 -> Switch/2
  TTC/1 -> 1-D Lookup Table/1
  1-D Lookup Table/1 -> Switch/3

== system acc_with_sensor_copy/Smooth Switch1/Smooth_Switch1 ==
  In1 : Inport
  Add : Sum
  Add1 : Sum  Inputs=+-
  Constant : Constant  Value=T/tau
  Constant1 : Constant
  Product : Product
  Product1 : Product
  Unit Delay : UnitDelay  InitialCondition=IC  SampleTime=T  HasFrameUpgradeWarning=on
  Out1 : Outport
  wires:
  Constant1/1 -> Add1/1
  Constant/1 -> Add1/2, Product1/2
  Add1/1 -> Product/1
  In1/1 -> Product1/1
  Product/1 -> Add/2
  Unit Delay/1 -> Product/2, Out1/1
  Add/1 -> Unit Delay/1
  Product1/1 -> Add/1

== system acc_with_sensor_copy/Subsystem/cut_off5 ==
  sign : Inport
  in : Inport  Port=2
  Delay : Delay  DelayLength=1  InitialConditionSource=Input port
      settings: InputPortMap=u0,p4
  Switch16 : Switch  Criteria=u2 ~= 0
  Out : Outport  VectorParamsAs1DForOutWhenUnconnected=off
  wires:
  in/1 -> Delay/2, Switch16/3
  sign/1 -> Switch16/2
  Switch16/1 -> Out/1, Delay/1
  Delay/1 -> Switch16/1

== system acc_with_sensor_copy/Subsystem2/Smooth_Switch1 ==
  In1 : Inport
  Add : Sum
  Add1 : Sum  Inputs=+-
  Constant : Constant  Value=T/tau
  Constant1 : Constant
  Product : Product
  Product1 : Product
  Unit Delay : UnitDelay  InitialCondition=IC  SampleTime=T  HasFrameUpgradeWarning=on
  Out1 : Outport
  wires:
  Constant1/1 -> Add1/1
  Constant/1 -> Add1/2, Product1/2
  Add1/1 -> Product/1
  In1/1 -> Product1/1
  Product/1 -> Add/2
  Unit Delay/1 -> Product/2, Out1/1
  Add/1 -> Unit Delay/1
  Product1/1 -> Add/1

== system acc_with_sensor_copy/Subsystem2/Smooth_Switch2 ==
  In1 : Inport
  Add : Sum
  Add1 : Sum  Inputs=+-
  Constant : Constant  Value=T/tau
  Constant1 : Constant
  Product : Product
  Product1 : Product
  Unit Delay : UnitDelay  InitialCondition=IC  SampleTime=T  HasFrameUpgradeWarning=on
  Out1 : Outport
  wires:
  Product1/1 -> Add/1
  Add/1 -> Unit Delay/1
  Unit Delay/1 -> Out1/1, Product/2
  Product/1 -> Add/2
  In1/1 -> Product1/1
  Add1/1 -> Product/1
  Constant/1 -> Product1/2, Add1/2
  Constant1/1 -> Add1/1

== system acc_with_sensor_copy/Subsystem4/rolling_avg1 ==
  note: Using the first two terms of the series expansion:
      |
      |                     x                     x2
      |                                e   =  1  +  x  +  --  + ......
      |                                           2!
      |
      |       Simplifying, the exponential "f" becomes:
      |
      |                  - (FK_TMR/TC)              1
      |           f  =  1  -  e                    =  1  -  -------------  =  . . .
      |                                                    (FK_TMR/TC)
      |                           e
      |
      |                              1                      1
      |          f  =  1  -  ---------------------------------  =    ------------------- .
      |                                  1 + (FK_TMR / TC)       1 + (TC / FK_TMR)
  note: - (FK_TMR/TC)
      |                                    f  =  1  -  e
      |
      |       Where "f" is called the filter constant in the difference equation:
      |
      |                    new_average = f * new_value + (1 - f) * old_average
  note: new_average = [ (sample_interval)/(sample_interval + time_constant) ] * (new_value - old_ave) + old_ave
  new_value : Inport
  old_ave : Inport  Port=2
  delta_t : Inport  Port=3
  tc : Inport  Port=4
  Divide : Product  Inputs=*/
  IC : UnitDelay  Tag=struct('comment',struct('text','','placement',1),'logdata',struct('maxnumvals',inf,'plotchannels',[],'stepsize',0,'downsampling',1,'loggingmode',3,'channels',1),'output',struct('width',1,'name','$S_$B','unit','','type','Int16','offset',0,'max',NaN,'min',NaN,'freeze',1,'lsb',1,'arb',0,'class','default','address','','description','','autoscalingmode',1,'lowerheadroom',1,'upperheadroom',1,'headroomunit','bit','checkmin',0,'checkmax',0,'show',0,'initial','2'),'state',0,'dt','-1','date',731455.586925799)  InitialCondition=1  SampleTime=0.1  HasFrameUpgradeWarning=on
  Interval Test : simulink/Logic and Bit Operations/Interval Test  IntervalClosedRight=on  uplimit=0.00001  IntervalClosedLeft=on  lowlimit=-0.00001  OutDataTypeStr=boolean
  Logical Operator : Logic  Operator=NOT  AllPortsSameDT=off  OutDataTypeStr=boolean
  Product_tmp1 : Product  Tag=struct('comment',struct('text','','placement',1),'logdata',struct('maxnumvals',inf,'plotchannels',[],'stepsize',0,'downsampling',1,'loggingmode',3,'channels',1),'output',struct('width',1,'name','$S_$B','unit','','type','Int32Bin15','offset',0,'max',65535,'min',-65536,'freeze',1,'lsb',2^-15,'arb',0,'class','default','address','','description','','autoscalingmode',1,'lowerheadroom',1,'upperheadroom',1,'headroomunit','bit','checkmin',0,'checkmax',0,'show',0),'inputs','**','exceptionhandling',1,'date',731455.58640515)  Inputs=**  InputSameDT=on  RndMeth=Zero  OutDataTypeStr=Inherit: Same as first input
  Sum : Sum  Tag=struct('comment',struct('text','','placement',1),'logdata',struct('maxnumvals',inf,'plotchannels',[],'stepsize',0,'downsampling',1,'loggingmode',3,'channels',1),'output',struct('width',1,'name','$S_$B','unit','','type','Int32Bin15','offset',0,'max',65535,'min',-65536,'freeze',1,'lsb',2^-15,'arb',0,'class','default','address','','description','','autoscalingmode',1,'lowerheadroom',1,'upperheadroom',1,'headroomunit','bit','checkmin',0,'checkmax',0,'show',0),'inputs','-+','date',731455.586330463)  Inputs=-+  InputSameDT=on  OutDataTypeStr=Inherit: Same as first input
  Sum1 : Sum  Tag=struct('comment',struct('text','','placement',1),'logdata',struct('maxnumvals',inf,'plotchannels',[],'stepsize',0,'downsampling',1,'loggingmode',3,'channels',1),'output',struct('width',1,'name','$S_$B','unit','','type','Int32Bin15','offset',0,'max',65535,'min',-65536,'freeze',1,'lsb',2^-15,'arb',0,'class','default','address','','description','','autoscalingmode',1,'lowerheadroom',1,'upperheadroom',1,'headroomunit','bit','checkmin',0,'checkmax',0,'show',0),'inputs','++','date',731455.58628235)  InputSameDT=on  OutDataTypeStr=Inherit: Same as first input
  Sum2 : Sum  Tag=struct('comment',struct('text','','placement',1),'logdata',struct('maxnumvals',inf,'plotchannels',[],'stepsize',0,'downsampling',1,'loggingmode',3,'channels',1),'output',struct('width',1,'name','$S_$B','unit','','type','Int32Bin15','offset',0,'max',65535,'min',-65536,'freeze',1,'lsb',2^-15,'arb',0,'class','default','address','','description','','autoscalingmode',1,'lowerheadroom',1,'upperheadroom',1,'headroomunit','bit','checkmin',0,'checkmax',0,'show',0),'inputs','++','date',731455.586506424)  InputSameDT=on  OutDataTypeStr=Inherit: Same as first input
  Switch : Switch  Criteria=u2 ~= 0
  Switch1 : Switch  Tag=struct('comment',struct('text','','placement',1),'logdata',struct('maxnumvals',inf,'plotchannels',[],'stepsize',0,'downsampling',1,'loggingmode',3,'channels',1),'output',struct('width',1,'name','$S_$B','unit','','type','Int32Bin15','offset',0,'max',65535,'min',-65536,'freeze',1,'lsb',2^-15,'arb',0,'class','default','address','','description','','autoscalingmode',1,'lowerheadroom',1,'upperheadroom',1,'headroomunit','bit','checkmin',0,'checkmax',0,'show',0),'threshold',struct('width',1,'name','$S_$B_threshold','unit','','type','Int16','offset',0,'max',NaN,'min',NaN,'freeze',1,'lsb',1,'arb',0,'class','default','address','','description','','value','1','scalar',0),'date',731455.58657044)  Threshold=0.5  InputSameDT=on
  zero : Constant  Tag=struct('comment',struct('text','','placement',1),'output',struct('width',1,'name','$S_$B','unit','','type','Int16','offset',0,'max',NaN,'min',NaN,'freeze',1,'lsb',1,'arb',0,'class','default','address','','description','','value','0','tolerance',1,'show',0),'date',731455.58675544)  Value=0  OutDataTypeStr=Inherit: Inherit via back propagation
  zero1 : Constant  Tag=struct('comment',struct('text','','placement',1),'output',struct('width',1,'name','$S_$B','unit','','type','Int16','offset',0,'max',NaN,'min',NaN,'freeze',1,'lsb',1,'arb',0,'class','default','address','','description','','value','0','tolerance',1,'show',0),'date',731455.58675544)  Value=0  OutDataTypeStr=Inherit: Inherit via back propagation
  new_ave : Outport
  wires:
  IC/1 -> Switch1/2
  Logical Operator/1 -> Switch/2
  Divide/1 -> Switch/1
  Interval Test/1 -> Logical Operator/1
  zero1/1 -> Switch/3
  Sum1/1 -> Divide/2, Interval Test/1
  old_ave/1 -> Sum2/1, Sum/1  "old_ave"
  zero/1 -> IC/1
  delta_t/1 -> Product_tmp1/2, Sum1/1  "delta_t"
  tc/1 -> Sum1/2
  Sum/1 -> Product_tmp1/1
  Switch1/1 -> new_ave/1  "new_ave"
  new_value/1 -> Sum/2, [new_value]  "new_value"
  Sum2/1 -> Switch1/3  "new_ave"
  [new_value] -> Switch1/1
  Product_tmp1/1 -> Divide/1
  Switch/1 -> Sum2/2

== system acc_with_sensor_copy/V_rel Estimation/Kalman filter ==
  cut_in_flg : Inport
  Jerk : Inport  Port=2
  S_rel : Inport  Port=3
  initial_value : Inport  Port=4
  Constant : Constant  Value=200  OutDataTypeStr=double
  Constant1 : Constant  Value=0.01  OutDataTypeStr=double
  Delay : Delay  DelayLength=1  InitialCondition=[1 0 0;0 1 0;0 0 1]  SampleTime=0.1
  Delay1 : Delay  DelayLength=1  InitialConditionSource=Input port  InitialCondition=[1;1;1]  ExternalReset=Rising  SampleTime=0.1
      settings: InputPortMap=u0,r5,p4
  Demux3 : Demux  Outputs=[1 1 1]
      settings: DisplayOption=none
  MATLAB Function2 : MATLAB Function  TreatAsAtomicUnit=on
  measurement update : MATLAB Function  TreatAsAtomicUnit=on
  time update : MATLAB Function  TreatAsAtomicUnit=on
  s_rel : Outport
  v_rel : Outport  Port=2
  a_rel : Outport  Port=3
  wires:
  S_rel/1 -> MATLAB Function2/3(Y)
  measurement update/1(X1) -> MATLAB Function2/1(X1)
  MATLAB Function2/1(X2) -> Demux3/1, Delay1/1
  Constant/1 -> time update/1(Q)
  initial_value/1 -> Delay1/3
  Delay/1 -> time update/3(M1)
  time update/2(M2) -> Delay/1
  Delay1/1 -> measurement update/1(X2)
  Constant1/1 -> time update/2(R)
  time update/1(K) -> MATLAB Function2/2(K)
  Demux3/1 -> s_rel/1
  Demux3/2 -> v_rel/1
  Demux3/3 -> a_rel/1
  Jerk/1 -> measurement update/2(u)
  cut_in_flg/1 -> Delay1/2

== system acc_with_sensor_copy/cmd_limiter1/rate_limit ==
  input_raw : Inport
  Sample_Time : Inport  Port=2
  ratelimt_incps : Inport  Port=3
  ratelimt_decps : Inport  Port=4
  Add : Sum  Inputs=+-
  Add1 : Sum
  Constant : Constant  Value=0  SampleTime=0.1
  Max : MinMax  Function=max  Inputs=2
  Max1 : MinMax  Inputs=2
  Max2 : MinMax  Function=max  Inputs=2
  Max3 : MinMax  Inputs=2
  Product : Product
  Product1 : Product
  Unit Delay : UnitDelay  SampleTime=0.1  HasFrameUpgradeWarning=on
  ax_cmd1 : Outport
  wires:
  Product1/1 -> Max2/1
  Product/1 -> Max3/2
  Sample_Time/1 -> Product/1, Product1/2
  ratelimt_incps/1 -> Product1/1
  ratelimt_decps/1 -> Product/2
  Constant/1 -> Max2/2, Max3/1
  Max3/1 -> [Dec]
  Max2/1 -> [Inc]
  Unit Delay/1 -> Add1/2, Add/2
  Add1/1 -> ax_cmd1/1, Unit Delay/1
  Max1/1 -> Add1/1
  [Dec] -> Max/2
  [Inc] -> Max1/1
  Max/1 -> Max1/2
  Add/1 -> Max/1
  input_raw/1 -> Add/1

== system acc_with_sensor_copy/cmd_limiter4/rate_limit ==
  input_raw : Inport
  Sample_Time : Inport  Port=2
  ratelimt_incps : Inport  Port=3
  ratelimt_decps : Inport  Port=4
  Add : Sum  Inputs=+-
  Add1 : Sum
  Constant : Constant  Value=0  SampleTime=0.1
  Max : MinMax  Function=max  Inputs=2
  Max1 : MinMax  Inputs=2
  Max2 : MinMax  Function=max  Inputs=2
  Max3 : MinMax  Inputs=2
  Product : Product
  Product1 : Product
  Unit Delay : UnitDelay  SampleTime=0.1  HasFrameUpgradeWarning=on
  ax_cmd1 : Outport
  wires:
  input_raw/1 -> Add/1
  Add/1 -> Max/1
  Max/1 -> Max1/2
  [Inc] -> Max1/1
  [Dec] -> Max/2
  Max1/1 -> Add1/1
  Add1/1 -> Unit Delay/1, ax_cmd1/1
  Unit Delay/1 -> Add/2, Add1/2
  Max2/1 -> [Inc]
  Max3/1 -> [Dec]
  Constant/1 -> Max3/1, Max2/2
  ratelimt_decps/1 -> Product/2
  ratelimt_incps/1 -> Product1/1
  Sample_Time/1 -> Product1/2, Product/1
  Product/1 -> Max3/2
  Product1/1 -> Max2/1

== matlab function acc_with_sensor_copy/Cut-in strategy/MATLAB Function11 ==
  data: tau input; u input; y output; old_u input
function y = fcn(tau,u,old_u)

T=0.1; % sample time

y=u*(T/(tau+T))+old_u*(tau/(tau+T));


end
